simulink model "swc_1"  (R2023b)
settings: Solver=FixedStepDiscrete  StartTime=0.0  StopTime=20.0  FixedStep=0.01  RelTol=1e-3
settings Model: TunableVars=auto_down_time,auto_up_time,emergency_down_time,position_endstop_top  TunableVarsStorageClass=Auto,Auto,Auto,Auto  TunableVarsTypeQualifier=,,,  Creator=Wolfgang Meincke  LastModifiedBy=developer
settings SolverCC: AlgebraicLoopSolver=TrustRegion
settings DataIOCC: LimitDataPoints=on  SaveFormat=Array  ReturnWorkspaceOutputs=off
settings OptimizationCC: BlockReduction=off  BooleanDataType=off  ConditionallyExecuteInputs=off  GlobalBufferReuse=off  EnableMemcpy=off  ExpressionDepthLimit=2147483647  ZeroExternalMemoryAtStartup=off  ZeroInternalMemoryAtStartup=off  InitFltsAndDblsToZero=on  NoFixptDivByZeroProtection=on  LifeSpan=1  EfficientTunableParamExpr=on
settings DebuggingCC: RTPrefix=none  SaveWithParameterizedLinksMsg=none  UnderspecifiedInitializationDetection=Classic  MergeDetectMultiDrivingBlocksExec=none  MultiTaskDSMMsg=warning  MultiTaskCondExecSysMsg=none  ParameterPrecisionLossMsg=none  FcnCallInpInsideContextMsg=warning  UnconnectedLineMsg=warning  AllowSymbolicDim=off  StateNameClashWarn=warning  SFUnexpectedBacktrackingDiag=warning  SFNoUnconditionalDefaultTransitionDiag=warning  SFExecutionAtInitializationDiag=none  ArithmeticOperatorsInVariantConditions=warning
settings HardwareCC: ProdLongLongMode=on
settings ModelReferenceCC: EnableRefExpFcnMdlSchedulingChecks=on  ModelReferenceNumInstancesAllowed=Single  PropagateSignalLabelsOutOfModel=off
settings SFSimCC: SimUseLocalCustomCode=off  SimParseCustomCode=off  MATLABDynamicMemAlloc=off  CustomCodeUndefinedFunction=UseInterfaceOnly
settings RTWCC: Description=Embedded Coder  SystemTargetFile=ert.tlc  GenCodeOnly=on  TemplateMakefile=ert_default_tmf  RetainRTWFile=on  RTWUseLocalCustomCode=off  Toolchain=MinGW64 | gmake (64-bit Windows)  PortableWordSizes=on
settings CodeAppCC: IgnoreCustomStorageClasses=off  MaxIdLength=40  StateflowObjectComments=on
settings ERTTargetCC: MultiwordLength=2048  IncludeMdlTerminateFcn=off  CombineSignalStateStructs=on  SupportAbsoluteTime=off  LogVarNameModifier=_rt  PurelyIntegerCode=on  SupportNonFinite=off  SupportComplex=off  RemoveResetFunc=off  RootIOFormat=Part of model data structure  ERTCustomFileTemplate=example_file_process.tlc  ConvertIfToSwitch=off  SuppressUnreachableDefaultCases=off
settings ConfigComp: CovMetricSettings=dw  CovSaveCumulativeToWorkspaceVar=on  CovSaveSingleToWorkspaceVar=on  CovExternalEMLEnable=off  CovSFcnEnable=off

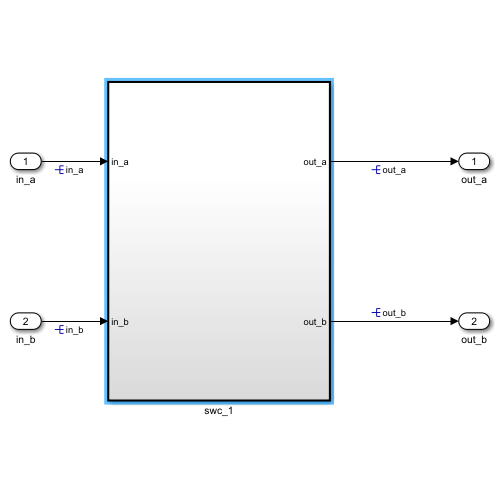
[thumbnail: Simulink's stored preview of the top-level diagram]
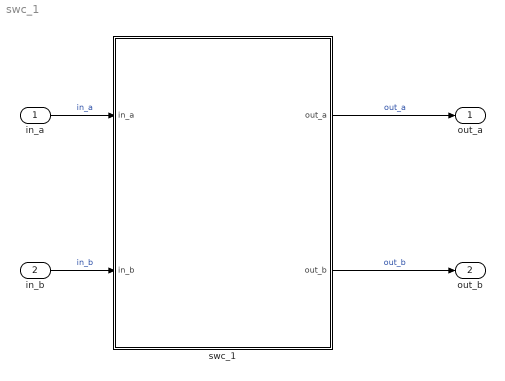
== system swc_1 ==
  in_a : Inport  OutMin=1  OutMax=199
  in_b : Inport  Port=2  OutMin=1  OutMax=199
  swc_1 : Subsystem  TreatAsAtomicUnit=on  RTWFcnName=swc_1_al
      settings: RTWSystemCode=Nonreusable function  RTWFcnNameOpts=User specified  RTWFileNameOpts=Use function name
  out_a : Outport  VectorParamsAs1DForOutWhenUnconnected=off
  out_b : Outport  Port=2  VectorParamsAs1DForOutWhenUnconnected=off
  wires:
  in_a/1 -> swc_1/1(in_a)  "in_a"
  in_b/1 -> swc_1/2(in_b)  "in_b"
  swc_1/1(out_a) -> out_a/1  "out_a"
  swc_1/2(out_b) -> out_b/1  "out_b"

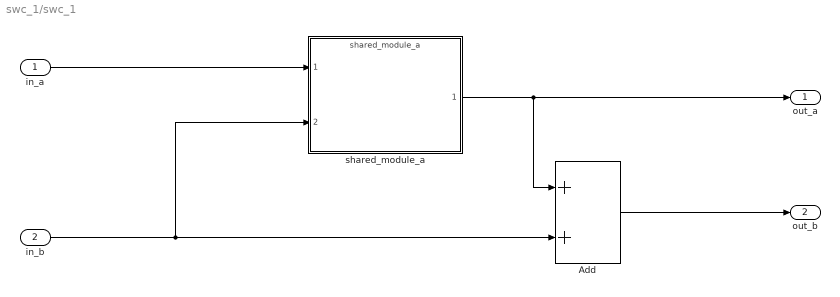
== system swc_1/swc_1 ==
  in_a : Inport  OutMin=1  OutMax=199
  in_b : Inport  Port=2  OutMin=1  OutMax=199
  Add : Sum
  shared_module_a : ModelReference  ModelNameDialog=shared_module_a.slx  SimulationMode=Normal  ModelReferenceVersion=3.1
  out_a : Outport  RequirementInfo={} %GIDa_cfaa6890_1b09_43c8_9181_c9775bd2e746  PortDimensions=1  VectorParamsAs1DForOutWhenUnconnected=off
  out_b : Outport  RequirementInfo={} %GIDa_e72b7e0a_8232_4793_901f_580fad4f0530  Port=2  PortDimensions=1  VectorParamsAs1DForOutWhenUnconnected=off
  wires:
  Add/1 -> out_b/1
  shared_module_a/1 -> Add/1, out_a/1
  in_b/1 -> shared_module_a/2, Add/2
  in_a/1 -> shared_module_a/1
